simulink model "SolarGrid"  (R2024b)
settings: Solver=VariableStepAuto  StartTime=0.0  StopTime=1  RelTol=1e-3
libraries: spsSeriesRLCBranchLib x18, spsMosfetLib x7, spsLinearTransformerLib x3, spsVoltageMeasurementLib x3, spsTriangleGeneratorLib x1, spsDiodeLib x1, spsPWMGeneratorDCDCLib x1, spsGroundLib x1, spsPVArrayLib x1, sps_lib x1
settings Model: Creator=Zidane Hadeed  LastModifiedBy=Zidane Hadeed

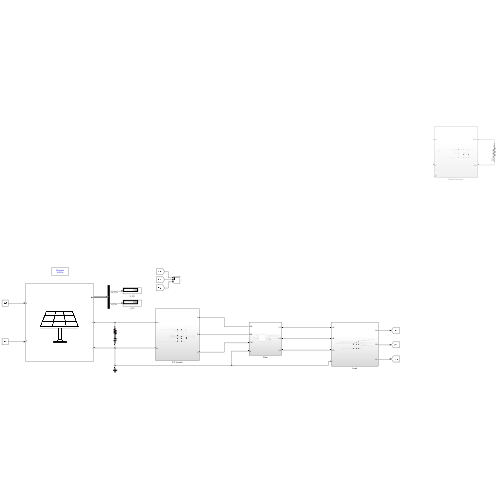
[thumbnail: Simulink's stored preview of the top-level diagram]
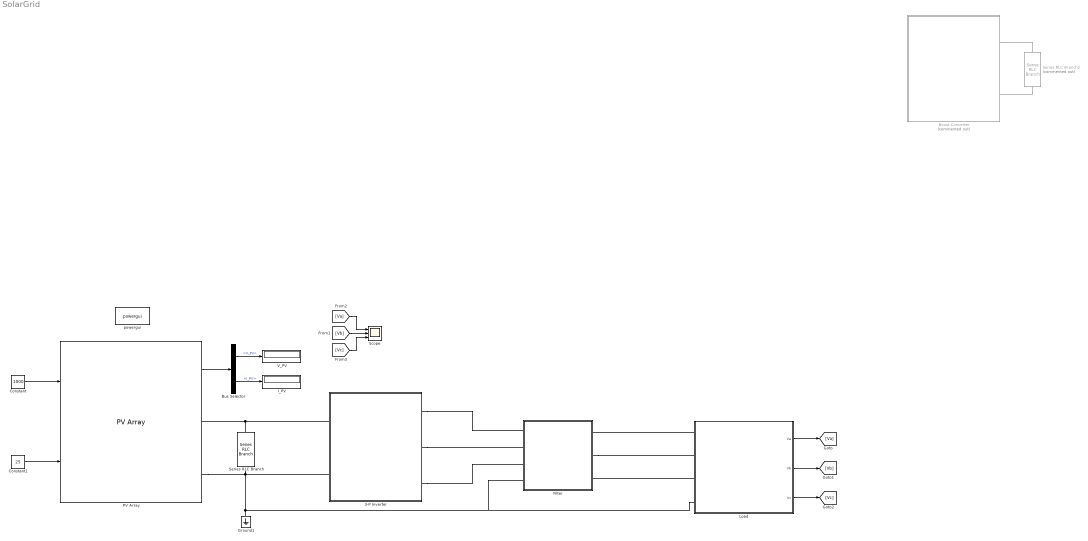
== system SolarGrid ==
  3-P Inverter : Subsystem
  Boost Converter : Subsystem  Commented=on
  Bus Selector : BusSelector  OutputSignals=V_PV,I_PV
  Constant : Constant  Value=1000
  Constant1 : Constant  Value=25
  Filter : Subsystem
  Ground1 : spsGroundLib/Ground  LConnTagsString=a
  I_PV : Display
  Load : Subsystem
  PV Array : spsPVArrayLib/PV Array  Npar=400  Nser=25  PlotType=array @ 25 deg.C & specified irradiances  S_vec="[ 1000  800  500 ]"  Temp_C_vec="[ 45 25  ]"  ModuleName=Amerisolar-Worldwide Energy and Manufacturing USA Co._ Ltd AS-6M-350W  PlotWhenSelected=off  Pm=350.0559  Ncell=72  Voc=47.64  Isc=9.59  Vm=38.51  Im=9.09  beta_Voc_pc=-0.297  alpha_Isc_pc=0.049103  beta_Voc=-0.14149  alpha_Isc=0.004709  IL=9.6509  I0=2.8976e-11  nI=0.97117  Rsh=367.1023  Rs=0.40738  RobustModel=off  RobustCellTemperature=313.3991  BAL=on  Tc=1e-6  Tfilter=5e-5
  Scope : Scope  NumInputPorts=3
  Series RLC Branch : spsSeriesRLCBranchLib/Series RLC Branch  LConnTagsString=__new0  RConnTagsString=__new0  BranchType=RC  Resistance=1e-2  Inductance=1e-3  SetiL0=off  InitialCurrent=0  Capacitance=4700e-6  Setx0=off  InitialVoltage=0  Measurements=None
  Series RLC Branch2 : spsSeriesRLCBranchLib/Series RLC Branch  Commented=on  LConnTagsString=__new0  RConnTagsString=__new0  BranchType=R  Resistance=10e3  Inductance=1e-3  SetiL0=off  InitialCurrent=0  Capacitance=1e-6  Setx0=off  InitialVoltage=0  Measurements=None
  V_PV : Display
  powergui : sps_lib/powergui  Priority=1  SimulationMode=Discrete  SampleTime=1e-6  frequency=60  Iterations=50  frequencyindice=0  Pbase=100e6  ErrMax=1e-4  UnitsV=kV  UnitsW=MW  buscounter=0  FunctionMessages=off  echomessages=off  EnableUseOfTLC=off  CurrentSourceSwitches=off  DisableSnubberDevices=off  DisableRonSwitches=off  DisableVfSwitches=off  DisplayEquations=off  AutomaticDiscreteSolvers=off  SolverType=Tustin/Backward Euler (TBE)  Interpol=off  ExternalGateDelay=off  methode=off  Ts=100  x0status=blocks  SPID=on  SwTol=0  HookPort=off  NonlinearTolerance=1e-4  nMaxIteration=100  ContinueOnMaxIteration=off  RestoreLinks=warning  ResistiveCurrentMeasurement=off  Frange=[0:2:500]  Ylog=off  Xlog=on  ShowGrid=off  save=off  variable=ZData  structure=0  ZoomFFT=off  StartTime=0.0  cycles=1  DisplayStyle=1  fundamental=60  FreqAxis=off  MaxFrequency=1000  frequencyindicesteady=1  RmsSteady=1  display=off
  wires:
  Constant/1 -> PV Array/1
  Constant1/1 -> PV Array/2
  [Va] -> Scope/1
  [Vb] -> Scope/2
  [Vc] -> Scope/3
  PV Array/1 -> Bus Selector/1
  Bus Selector/1 -> V_PV/1  "<V_PV>"
  Bus Selector/2 -> I_PV/1  "<I_PV>"
  Load/1(Va) -> [Va]
  Load/2(Vb) -> [Vb]
  Load/3(Vc) -> [Vc]
  connections:
  Series RLC Branch/LConn1 -- 3-P Inverter/LConn1 -- PV Array/RConn1
  Boost Converter/RConn1 -- Series RLC Branch2/RConn1
  Series RLC Branch2/LConn1 -- Boost Converter/RConn2
  3-P Inverter/LConn2 -- Filter/LConn4 -- Load/LConn4 -- Ground1/LConn1 -- PV Array/RConn2 -- Series RLC Branch/RConn1
  3-P Inverter/RConn1 -- Filter/LConn1
  Load/LConn1 -- Filter/RConn1
  Filter/RConn2 -- Load/LConn2
  3-P Inverter/RConn2 -- Filter/LConn2
  Load/LConn3 -- Filter/RConn3
  3-P Inverter/RConn3 -- Filter/LConn3

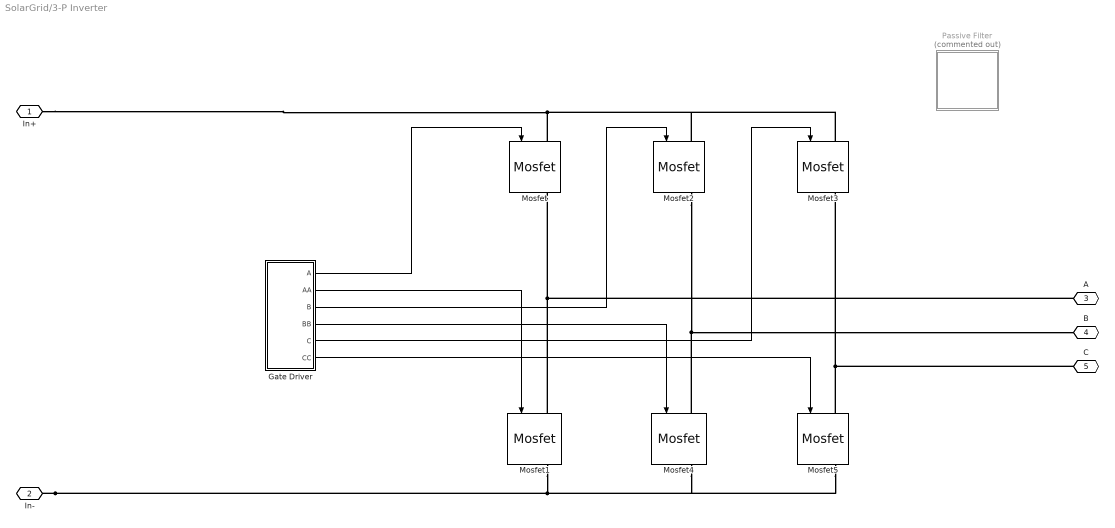
== system SolarGrid/3-P Inverter ==
  Gate Driver : Subsystem
  Mosfet{,1..5} (6 alike) : spsMosfetLib/Mosfet  Ron=0.1  Lon=0  Rd=0.01  Vfd=0  IC=0  Rs=1e5  Cs=inf  Measurements=on
  Passive Filter : Subsystem  Commented=on
      settings: PortSchema="{\"entries\":[{\"content\":{\"sides\":[{\"content\":{\"connectorIds\":[\"LConn1\",\"LConn2\",\"LConn3\"]},\"type\":\"ConnectorPlacement.EquallySpacedRectSide\",\"uuid\":\"62e55c9e-b411-4f10-a29f-aa0c5be36897\"},{\"content\":{\"connectorIds\":[\"RConn1\",\"RConn2\",\"RConn3\"],\"side\":\"RIGHT\"},\"type\":\"ConnectorPlacement.EquallySpacedRectSide\",\"uuid\":\"476f1a27-74f2-436a-8fc3-e2e5d83bb21b\"},{\"content\":{\"side\":\"TOP\"},\"type\":\"ConnectorPlacement.EquallySpacedRectSide\",\"uuid\":\"6a538d83-3a6b-4d9f-b9e9-43834189a8fd\"},{\"content\":{\"connectorIds\":[\"RConn4\"],\"side\":\"BOTTOM\"},\"type\":\"ConnectorPlacement.EquallySpacedRectSide\",\"uuid\":\"d798d2e6-cd10-429f-9f9b-8383104bce78\"}]},\"type\":\"ConnectorPlacement.EquallySpacedConnector\",\"uuid\":\"0b9f9509-cccf-4838-84a5-b9f3e67ee63a\"}],\"packageUris\":[\"http://schema.mathworks.com/mf0/Connector/R2020b\"],\"version\":\"1.0\"}"
  In+ : PMIOPort  Side=Left
  In- : PMIOPort  Port=2  Side=Left
  A : PMIOPort  Port=3  Side=Right
  B : PMIOPort  Port=4  Side=Right
  C : PMIOPort  Port=5  Side=Right
  wires:
  Gate Driver/1(A) -> Mosfet/1
  Gate Driver/2(AA) -> Mosfet1/1
  Gate Driver/3(B) -> Mosfet2/1
  Gate Driver/4(BB) -> Mosfet4/1
  Gate Driver/5(C) -> Mosfet3/1
  Gate Driver/6(CC) -> Mosfet5/1
  connections:
  In-/RConn1 -- Mosfet5/RConn1 -- Mosfet4/RConn1 -- Mosfet1/RConn1
  In+/RConn1 -- Mosfet3/LConn1 -- Mosfet2/LConn1 -- Mosfet/LConn1
  Mosfet5/LConn1 -- Mosfet3/RConn1 -- C/RConn1
  Mosfet1/LConn1 -- Mosfet/RConn1 -- A/RConn1
  Mosfet2/RConn1 -- Mosfet4/LConn1 -- B/RConn1

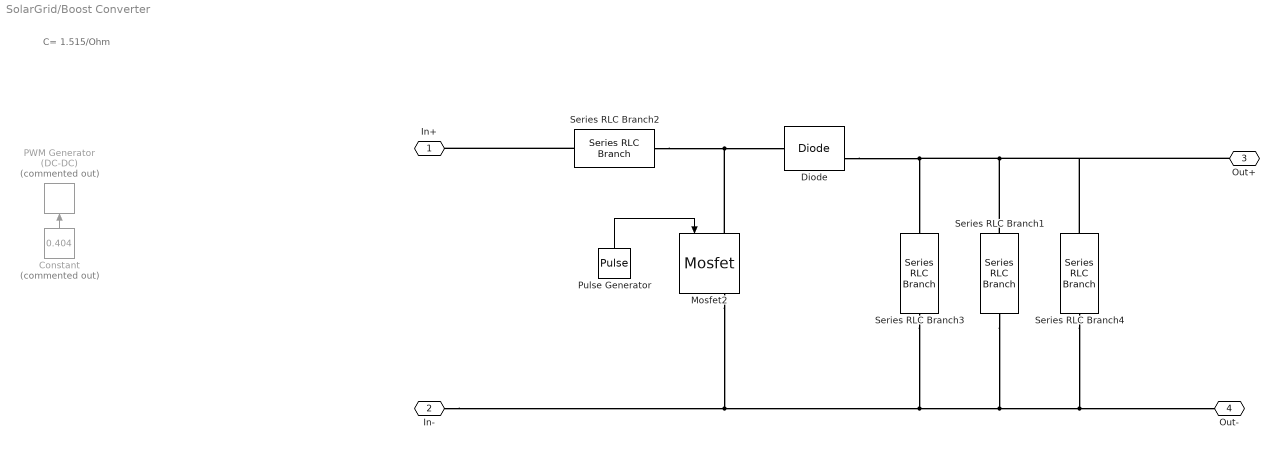
== system SolarGrid/Boost Converter ==
  note: C= 1.515/Ohm
  Constant : Constant  Commented=on  Value=0.404
  Diode : spsDiodeLib/Diode  Ron=0.001  Lon=0  Vf=0.8  IC=0  UseSnubber=0  Rs=500  Cs=250e-9  Measurements=on
  Mosfet2 : spsMosfetLib/Mosfet  Ron=0.1  Lon=0  Rd=0.01  Vfd=0  IC=0  Rs=1e5  Cs=inf  Measurements=on
  PWM Generator (DC-DC) : spsPWMGeneratorDCDCLib/PWM Generator (DC-DC)  Commented=on  Fsw=10000  Ts=0
  Pulse Generator : DiscretePulseGenerator  PulseType=Time based  Period=1/10e3  PulseWidth=90
  Series RLC Branch1 : spsSeriesRLCBranchLib/Series RLC Branch  LConnTagsString=__new0  RConnTagsString=__new0  BranchType=RC  Resistance=1e-2  Inductance=1e-3  SetiL0=off  InitialCurrent=0  Capacitance=4700e-6  Setx0=off  InitialVoltage=0  Measurements=None
  Series RLC Branch2 : spsSeriesRLCBranchLib/Series RLC Branch  LConnTagsString=__new0  RConnTagsString=__new0  BranchType=L  Resistance=1e-2  Inductance=900e-3  SetiL0=off  InitialCurrent=0  Capacitance=10e-6  Setx0=off  InitialVoltage=0  Measurements=None
  Series RLC Branch3 : spsSeriesRLCBranchLib/Series RLC Branch  LConnTagsString=__new0  RConnTagsString=__new0  BranchType=RC  Resistance=1e-2  Inductance=1e-3  SetiL0=off  InitialCurrent=0  Capacitance=4700e-6  Setx0=off  InitialVoltage=0  Measurements=None
  Series RLC Branch4 : spsSeriesRLCBranchLib/Series RLC Branch  LConnTagsString=__new0  RConnTagsString=__new0  BranchType=RC  Resistance=1e-2  Inductance=1e-3  SetiL0=off  InitialCurrent=0  Capacitance=4700e-6  Setx0=off  InitialVoltage=0  Measurements=None
  In+ : PMIOPort  Side=Left
  In- : PMIOPort  Port=2  Side=Left
  Out+ : PMIOPort  Port=3  Side=Right
  Out- : PMIOPort  Port=4  Side=Right
  wires:
  Constant/1 -> PWM Generator (DC-DC)/1
  Pulse Generator/1 -> Mosfet2/1
  connections:
  Series RLC Branch2/LConn1 -- Mosfet2/LConn1 -- Diode/LConn1
  Diode/RConn1 -- Series RLC Branch4/LConn1 -- Out+/RConn1 -- Series RLC Branch1/LConn1 -- Series RLC Branch3/LConn1
  In-/RConn1 -- Mosfet2/RConn1 -- Series RLC Branch3/RConn1 -- Series RLC Branch1/RConn1 -- Series RLC Branch4/RConn1 -- Out-/RConn1
  Series RLC Branch2/RConn1 -- In+/RConn1

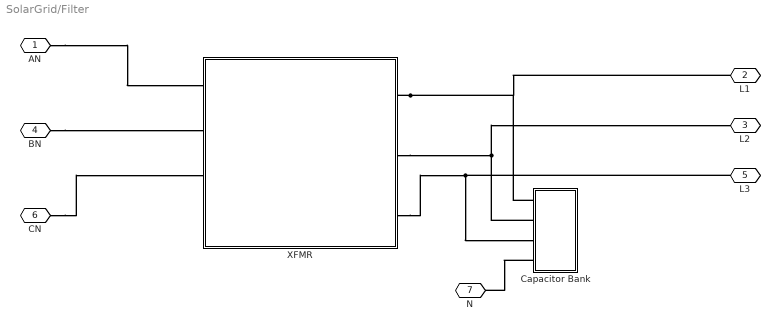
== system SolarGrid/Filter ==
  Capacitor Bank : Subsystem
  XFMR : Subsystem
  AN : PMIOPort  Side=Left
  L1 : PMIOPort  Port=2  Side=Right
  L2 : PMIOPort  Port=3  Side=Right
  BN : PMIOPort  Port=4  Side=Left
  L3 : PMIOPort  Port=5  Side=Right
  CN : PMIOPort  Port=6  Side=Left
  N : PMIOPort  Port=7  Side=Left
  connections:
  XFMR/RConn2 -- L2/RConn1 -- Capacitor Bank/LConn2
  XFMR/RConn1 -- L1/RConn1 -- Capacitor Bank/LConn1
  CN/RConn1 -- XFMR/LConn3
  XFMR/RConn3 -- L3/RConn1 -- Capacitor Bank/LConn3
  Capacitor Bank/LConn4 -- N/RConn1
  BN/RConn1 -- XFMR/LConn2
  AN/RConn1 -- XFMR/LConn1

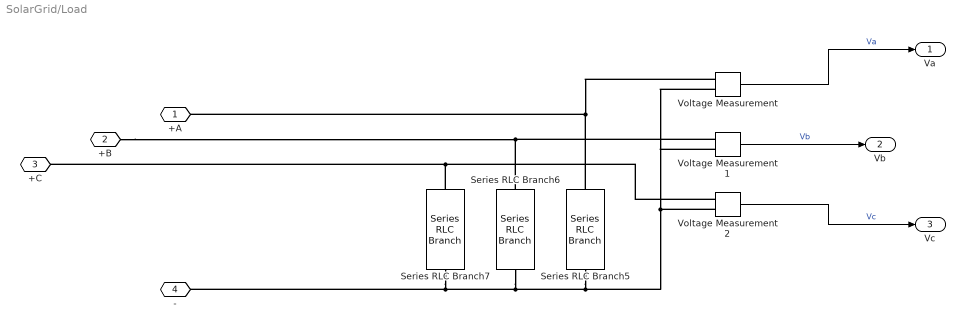
== system SolarGrid/Load ==
  Series RLC Branch5 : spsSeriesRLCBranchLib/Series RLC Branch  LConnTagsString=__new0  RConnTagsString=__new0  BranchType=R  Resistance=1e3  Inductance=1e-3  SetiL0=off  InitialCurrent=0  Capacitance=1e-6  Setx0=off  InitialVoltage=0  Measurements=None
  Series RLC Branch6 : spsSeriesRLCBranchLib/Series RLC Branch  LConnTagsString=__new0  RConnTagsString=__new0  BranchType=R  Resistance=1e3  Inductance=1e-3  SetiL0=off  InitialCurrent=0  Capacitance=1e-6  Setx0=off  InitialVoltage=0  Measurements=None
  Series RLC Branch7 : spsSeriesRLCBranchLib/Series RLC Branch  LConnTagsString=__new0  RConnTagsString=__new0  BranchType=R  Resistance=1e3  Inductance=1e-3  SetiL0=off  InitialCurrent=0  Capacitance=1e-6  Setx0=off  InitialVoltage=0  Measurements=None
  Voltage Measurement : spsVoltageMeasurementLib/Voltage Measurement  PhasorSimulation=off  OutputType=Complex  PSBequivalent=0
  Voltage Measurement1 : spsVoltageMeasurementLib/Voltage Measurement  PhasorSimulation=off  OutputType=Complex  PSBequivalent=0
  Voltage Measurement2 : spsVoltageMeasurementLib/Voltage Measurement  PhasorSimulation=off  OutputType=Complex  PSBequivalent=0
  +A : PMIOPort  Side=Left
  +B : PMIOPort  Port=2  Side=Left
  +C : PMIOPort  Port=3  Side=Left
  - : PMIOPort  Port=4  Side=Left
  Va : Outport
  Vb : Outport  Port=2
  Vc : Outport  Port=3
  wires:
  Voltage Measurement/1 -> Va/1  "Va"
  Voltage Measurement2/1 -> Vc/1  "Vc"
  Voltage Measurement1/1 -> Vb/1  "Vb"
  connections:
  Series RLC Branch7/LConn1 -- +C/RConn1 -- Voltage Measurement2/LConn1
  Series RLC Branch7/RConn1 -- -/RConn1 -- Voltage Measurement1/LConn2 -- Voltage Measurement/LConn2 -- Voltage Measurement2/LConn2 -- Series RLC Branch5/RConn1 -- Series RLC Branch6/RConn1
  Voltage Measurement1/LConn1 -- Series RLC Branch6/LConn1 -- +B/RConn1
  Voltage Measurement/LConn1 -- +A/RConn1 -- Series RLC Branch5/LConn1

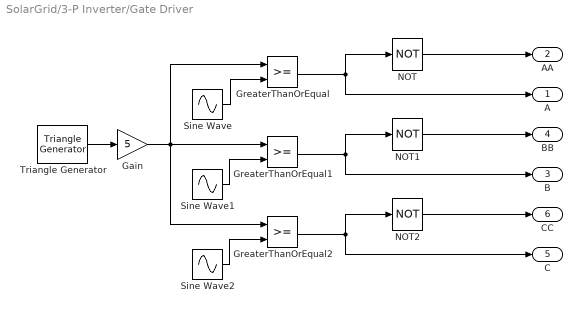
== system SolarGrid/3-P Inverter/Gate Driver ==
  Gain : Gain  Gain=5
  GreaterThanOrEqual : RelationalOperator  OutDataTypeStr=boolean  RndMeth=Simplest  InputSameDT=off
  GreaterThanOrEqual1 : RelationalOperator  OutDataTypeStr=boolean  RndMeth=Simplest  InputSameDT=off
  GreaterThanOrEqual2 : RelationalOperator  OutDataTypeStr=boolean  RndMeth=Simplest  InputSameDT=off
  NOT : Logic  Operator=NOT  IconShape=distinctive  AllPortsSameDT=off  OutDataTypeStr=boolean
  NOT1 : Logic  Operator=NOT  IconShape=distinctive  AllPortsSameDT=off  OutDataTypeStr=boolean
  NOT2 : Logic  Operator=NOT  IconShape=distinctive  AllPortsSameDT=off  OutDataTypeStr=boolean
  Sine Wave : Sin  Amplitude=5  Frequency=100*pi  SampleTime=0
  Sine Wave1 : Sin  Amplitude=5  Frequency=100*pi  Phase=2*pi/3  SampleTime=0
  Sine Wave2 : Sin  Amplitude=5  Frequency=100*pi  Phase=4*pi/3  SampleTime=0
  Triangle Generator : spsTriangleGeneratorLib/Triangle Generator  Freq=300  Phase=0  Ts=0
  A : Outport
  AA : Outport  Port=2
  B : Outport  Port=3
  BB : Outport  Port=4
  C : Outport  Port=5
  CC : Outport  Port=6
  wires:
  GreaterThanOrEqual1/1 -> B/1, NOT1/1
  Sine Wave1/1 -> GreaterThanOrEqual1/2
  Triangle Generator/1 -> Gain/1
  Sine Wave2/1 -> GreaterThanOrEqual2/2
  Sine Wave/1 -> GreaterThanOrEqual/2
  NOT1/1 -> BB/1
  Gain/1 -> GreaterThanOrEqual2/1, GreaterThanOrEqual1/1, GreaterThanOrEqual/1
  NOT/1 -> AA/1
  GreaterThanOrEqual2/1 -> C/1, NOT2/1
  GreaterThanOrEqual/1 -> NOT/1, A/1
  NOT2/1 -> CC/1

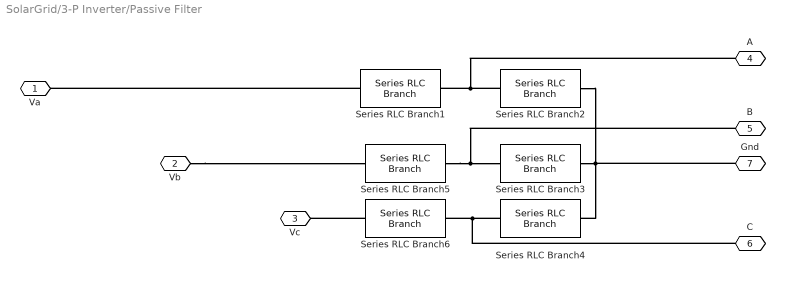
== system SolarGrid/3-P Inverter/Passive Filter ==
  Series RLC Branch1 : spsSeriesRLCBranchLib/Series RLC Branch  LConnTagsString=__new0  RConnTagsString=__new0  BranchType=L  Resistance=1  Inductance=100e-3  SetiL0=off  InitialCurrent=0  Capacitance=540e-3  Setx0=off  InitialVoltage=0  Measurements=None
  Series RLC Branch2 : spsSeriesRLCBranchLib/Series RLC Branch  LConnTagsString=__new0  RConnTagsString=__new0  BranchType=C  Resistance=1  Inductance=1e-3  SetiL0=off  InitialCurrent=0  Capacitance=100e-6  Setx0=off  InitialVoltage=0  Measurements=None
  Series RLC Branch3 : spsSeriesRLCBranchLib/Series RLC Branch  LConnTagsString=__new0  RConnTagsString=__new0  BranchType=C  Resistance=1  Inductance=1e-3  SetiL0=off  InitialCurrent=0  Capacitance=100e-6  Setx0=off  InitialVoltage=0  Measurements=None
  Series RLC Branch4 : spsSeriesRLCBranchLib/Series RLC Branch  LConnTagsString=__new0  RConnTagsString=__new0  BranchType=C  Resistance=1  Inductance=1e-3  SetiL0=off  InitialCurrent=0  Capacitance=100e-6  Setx0=off  InitialVoltage=0  Measurements=None
  Series RLC Branch5 : spsSeriesRLCBranchLib/Series RLC Branch  LConnTagsString=__new0  RConnTagsString=__new0  BranchType=L  Resistance=1  Inductance=100e-3  SetiL0=off  InitialCurrent=0  Capacitance=540e-3  Setx0=off  InitialVoltage=0  Measurements=None
  Series RLC Branch6 : spsSeriesRLCBranchLib/Series RLC Branch  LConnTagsString=__new0  RConnTagsString=__new0  BranchType=L  Resistance=1  Inductance=100e-3  SetiL0=off  InitialCurrent=0  Capacitance=540e-3  Setx0=off  InitialVoltage=0  Measurements=None
  Va : PMIOPort  Side=Left
  Vb : PMIOPort  Port=2  Side=Left
  Vc : PMIOPort  Port=3  Side=Left
  A : PMIOPort  Port=4  Side=Right
  B : PMIOPort  Port=5  Side=Right
  C : PMIOPort  Port=6  Side=Right
  Gnd : PMIOPort  Port=7  Side=Right
  connections:
  Series RLC Branch4/LConn1 -- C/RConn1 -- Series RLC Branch6/RConn1
  B/RConn1 -- Series RLC Branch3/LConn1 -- Series RLC Branch5/RConn1
  Series RLC Branch1/LConn1 -- Va/RConn1
  Series RLC Branch2/RConn1 -- Gnd/RConn1 -- Series RLC Branch3/RConn1 -- Series RLC Branch4/RConn1
  Series RLC Branch2/LConn1 -- Series RLC Branch1/RConn1 -- A/RConn1
  Vb/RConn1 -- Series RLC Branch5/LConn1
  Series RLC Branch6/LConn1 -- Vc/RConn1

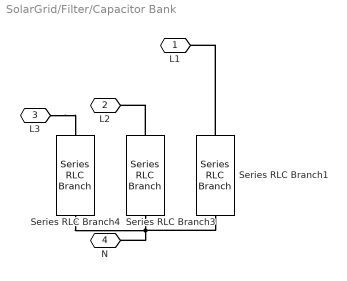
== system SolarGrid/Filter/Capacitor Bank ==
  Series RLC Branch1 : spsSeriesRLCBranchLib/Series RLC Branch  LConnTagsString=__new0  RConnTagsString=__new0  BranchType=C  Resistance=1  Inductance=1e-3  SetiL0=off  InitialCurrent=0  Capacitance=10e-6  Setx0=off  InitialVoltage=0  Measurements=None
  Series RLC Branch3 : spsSeriesRLCBranchLib/Series RLC Branch  LConnTagsString=__new0  RConnTagsString=__new0  BranchType=C  Resistance=1  Inductance=1e-3  SetiL0=off  InitialCurrent=0  Capacitance=10e-6  Setx0=off  InitialVoltage=0  Measurements=None
  Series RLC Branch4 : spsSeriesRLCBranchLib/Series RLC Branch  LConnTagsString=__new0  RConnTagsString=__new0  BranchType=C  Resistance=1  Inductance=1e-3  SetiL0=off  InitialCurrent=0  Capacitance=10e-6  Setx0=off  InitialVoltage=0  Measurements=None
  L1 : PMIOPort  Side=Left
  L2 : PMIOPort  Port=2  Side=Left
  L3 : PMIOPort  Port=3  Side=Left
  N : PMIOPort  Port=4  Side=Left
  connections:
  L3/RConn1 -- Series RLC Branch4/LConn1
  Series RLC Branch1/RConn1 -- N/RConn1 -- Series RLC Branch4/RConn1 -- Series RLC Branch3/RConn1
  Series RLC Branch3/LConn1 -- L2/RConn1
  Series RLC Branch1/LConn1 -- L1/RConn1

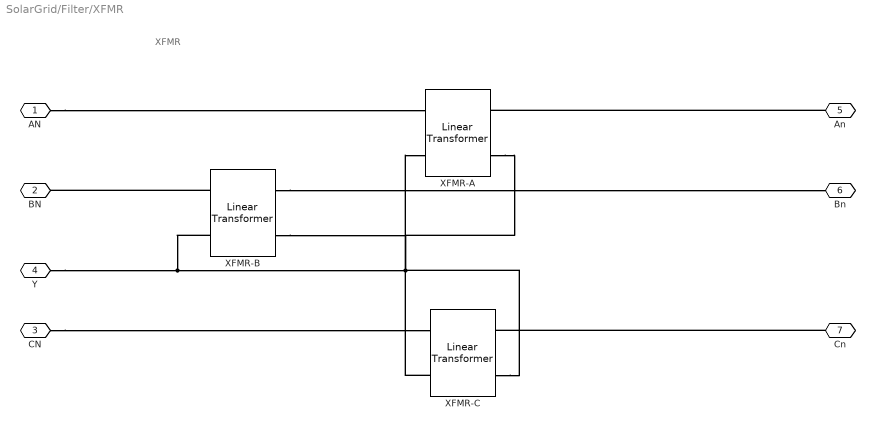
== system SolarGrid/Filter/XFMR ==
  note: XFMR
  XFMR-A : spsLinearTransformerLib/Linear Transformer  UNITS=SI  NominalPower=[ 250e6 60 ]  winding1=[3.15e+05 0.7938 0.084225]  winding2=[7.35e+05 4.3218 0.45856]  ThreeWindings=off  winding3=[3.15e+05 0.7938 0.084225]  RmLm=[1.0804e+06 2866]  Measurements=All voltages and currents  DataType=on
  XFMR-B : spsLinearTransformerLib/Linear Transformer  UNITS=SI  NominalPower=[ 250e6 60 ]  winding1=[3.15e+05 0.7938 0.084225]  winding2=[7.35e+05 4.3218 0.45856]  ThreeWindings=off  winding3=[3.15e+05 0.7938 0.084225]  RmLm=[1.0804e+06 2866]  Measurements=All voltages and currents  DataType=on
  XFMR-C : spsLinearTransformerLib/Linear Transformer  UNITS=SI  NominalPower=[ 250e6 60 ]  winding1=[3.15e+05 0.7938 0.084225]  winding2=[7.35e+05 4.3218 0.45856]  ThreeWindings=off  winding3=[3.15e+05 0.7938 0.084225]  RmLm=[1.0804e+06 2866]  Measurements=All voltages and currents  DataType=on
  AN : PMIOPort  Side=Left
  BN : PMIOPort  Port=2  Side=Left
  CN : PMIOPort  Port=3  Side=Left
  Y : PMIOPort  Port=4  Side=Left
  An : PMIOPort  Port=5  Side=Right
  Bn : PMIOPort  Port=6  Side=Right
  Cn : PMIOPort  Port=7  Side=Right
  connections:
  XFMR-B/LConn2 -- XFMR-C/LConn2 -- XFMR-C/RConn2 -- XFMR-A/RConn2 -- XFMR-B/RConn2 -- XFMR-A/LConn2 -- Y/RConn1
  AN/RConn1 -- XFMR-A/LConn1
  XFMR-B/LConn1 -- BN/RConn1
  An/RConn1 -- XFMR-A/RConn1
  XFMR-B/RConn1 -- Bn/RConn1
  Cn/RConn1 -- XFMR-C/RConn1
  CN/RConn1 -- XFMR-C/LConn1
